simulink model "T15_DD"  (R2018a)
settings: configuration reference "cs_ert" (kept outside this file)
model workspace (MAT data in the model file):
  T15_DD_DT = 10
values from neighbouring files (symbols this model uses):
  T15_tiDebHiLo_C = 10.0    [T15_DD.sldd]
  T15_tiDebLoHi_C = 10.0    [T15_DD.sldd]
  T15_uThreshold_C = 800.0    [T15_DD.sldd]
libraries: sllib x1
settings Model: DataDictionary=T15_DD.sldd  Creator=zhoutinglin  LastModifiedBy=zhoutinglin

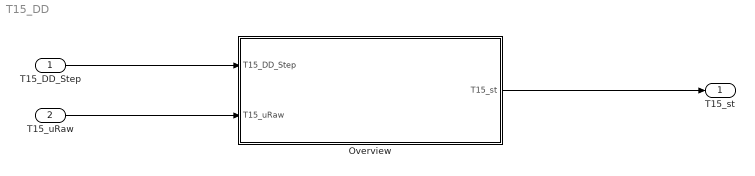
== system T15_DD ==
  T15_DD_Step : Inport  OutputFunctionCall=on
  T15_uRaw : Inport  Description=Raw ADC value of downstream engine coolant temperature sensor signal  Port=2  OutMin=0  OutMax=5000  OutDataTypeStr=Volt_mV  Unit=mv  PortDimensions=[1 1]
  Overview : Subsystem
  T15_st : Outport  Description=Terminal 15 status after debouncing  OutDataTypeStr=Enum:Switch  PortDimensions=[1 1]
  wires:
  T15_DD_Step/1 -> Overview/1(T15_DD_Step)
  T15_uRaw/1 -> Overview/2(T15_uRaw)
  Overview/1(T15_st) -> T15_st/1

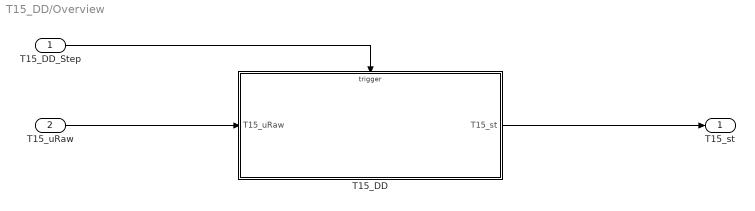
== system T15_DD/Overview ==
  T15_DD_Step : Inport
  T15_uRaw : Inport  Port=2
  T15_DD : Subsystem
  T15_st : Outport
  wires:
  T15_uRaw/1 -> T15_DD/1(T15_uRaw)
  T15_DD/1(T15_st) -> T15_st/1
  T15_DD_Step/1 -> T15_DD/Trigger

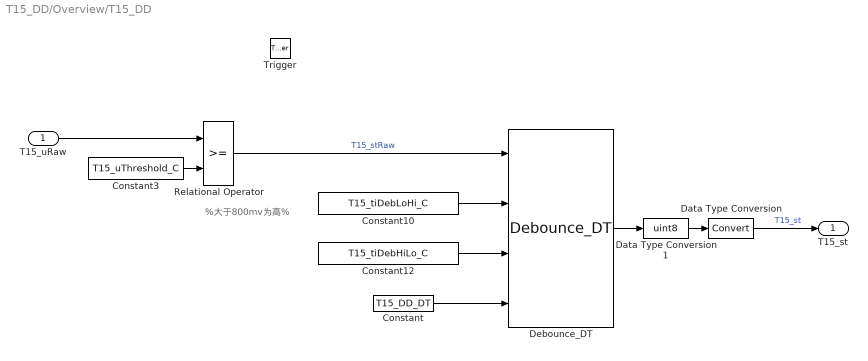
== system T15_DD/Overview/T15_DD ==
  note: %大于800mv为高%
  T15_uRaw : Inport  Tag=mv
  Trigger : TriggerPort  TriggerType=function-call  VariantControl=Variant  PortDimensions=1
  Constant : Constant  Value=T15_DD_DT  OutDataTypeStr=Inherit: Inherit via back propagation
  Constant10 : Constant  Value=T15_tiDebLoHi_C
  Constant12 : Constant  Value=T15_tiDebHiLo_C
  Constant3 : Constant  Value=T15_uThreshold_C
  Data Type Conversion : DataTypeConversion
  Data Type Conversion1 : DataTypeConversion  OutDataTypeStr=uint8
  Debounce_DT : sllib/Debounce_DT
      settings: SourceProductName=sllib
  Relational Operator : RelationalOperator  OutDataTypeStr=boolean  RndMeth=Nearest  InputSameDT=on
  T15_st : Outport
  wires:
  Constant3/1 -> Relational Operator/2
  Constant12/1 -> Debounce_DT/3
  Relational Operator/1 -> Debounce_DT/1  "T15_stRaw"
  Data Type Conversion/1 -> T15_st/1  "T15_st"
  Data Type Conversion1/1 -> Data Type Conversion/1
  T15_uRaw/1 -> Relational Operator/1
  Constant/1 -> Debounce_DT/4
  Constant10/1 -> Debounce_DT/2
  Debounce_DT/1 -> Data Type Conversion1/1
